simulink model "shipmodel5446"  (Simulink 8.3)
settings: Solver=ode3  StartTime=0.0  StopTime=600  FixedStep=0.3  RelTol=1e-3
libraries: simulink x1
settings Model: Creator=Administrator  LastModifiedBy=hasee
settings OptimizationCC: ExpressionDepthLimit=2147483647
settings DebuggingCC: FcnCallInpInsideContextMsg=UseLocalSettings

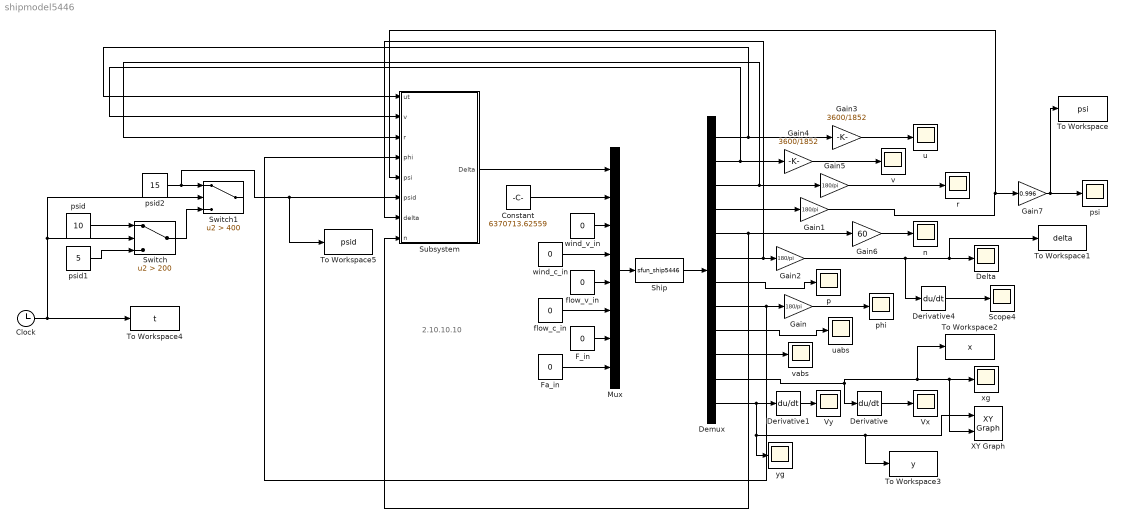
== system shipmodel5446 ==
  note: 2.10.10.10
  Clock : Clock
  Constant : Constant  Value=6370713.62559
  Delta : Scope
      settings: TickLabels=on  TimeRange=600  YMin=-2.5  YMax=25  SaveName=ScopeData5
  Demux : Demux  Outputs=12
  Derivative : Derivative
  Derivative1 : Derivative
  Derivative4 : Derivative
  F_in : Constant  Value=0
  Fa_in : Constant  Value=0
  Gain{,1..2,5} (4 alike) : Gain  Gain=180/pi
  Gain3 : Gain  Gain=3600/1852
  Gain4 : Gain  Gain=3600/1852
  Gain6 : Gain  Gain=60
  Gain7 : Gain  Gain=0.996
  Mux : Mux  Inputs=8
  Scope4 : Scope
      settings: YMin=-3  YMax=3  SaveName=ScopeData18
  Ship : S-Function  FunctionName=sfun_ship5446  EnableBusSupport=off
  Subsystem : Subsystem
  Switch : Switch  Criteria=u2 > Threshold  Threshold=200
  Switch1 : Switch  Criteria=u2 > Threshold  Threshold=400
  To Workspace : ToWorkspace  VariableName=psi  SampleTime=-1
  To Workspace1 : ToWorkspace  VariableName=delta  SampleTime=-1
  To Workspace2 : ToWorkspace  VariableName=x  SampleTime=-1
  To Workspace3 : ToWorkspace  VariableName=y  SampleTime=-1
  To Workspace4 : ToWorkspace  VariableName=t  SampleTime=-1
  To Workspace5 : ToWorkspace  VariableName=psid  SampleTime=-1
  Vx : Scope
      settings: TickLabels=on  SaveName=ScopeData8
  Vy : Scope
      settings: TickLabels=on  SaveName=ScopeData9
  XY Graph : simulink/Sinks/XY Graph  xmin=-2000  xmax=2000  ymin=-200  ymax=4500  st=-1
  flow_c_in : Constant  Value=0
  flow_v_in : Constant  Value=0
  n : Scope
      settings: TickLabels=on  YMin=99.475  YMax=99.8  SaveName=ScopeData4
  p : Scope
      settings: TickLabels=on  SaveName=ScopeData10
  phi : Scope
      settings: YMin=-0.175  YMax=0.125  SaveName=ScopeData11
  psi : Scope
      settings: TickLabels=on  TimeRange=600  YMin=0  YMax=16  SaveName=ScopeData3
  psid : Constant  Value=10
  psid1 : Constant  Value=5
  psid2 : Constant  Value=15
  r : Scope
      settings: TickLabels=on  SaveName=ScopeData2
  u : Scope
      settings: TickLabels=on  YMin=27.45  YMax=28.35
  uabs : Scope
      settings: TickLabels=on  YMin=10.75  YMax=15  SaveName=ScopeData6
  v : Scope
      settings: TickLabels=on  YMin=-0.0975  YMax=-0.055
  vabs : Scope
      settings: TickLabels=on  YMin=-1.75  YMax=0  SaveName=ScopeData7
  wind_c_in : Constant  Value=0
  wind_v_in : Constant  Value=0
  xg : Scope
      settings: TickLabels=on  YMin=250  YMax=475  SaveName=ScopeData12
  yg : Scope
      settings: TickLabels=on  YMin=250  YMax=475  SaveName=ScopeData13
  wires:
  Ship/1 -> Demux/1
  Demux/1 -> Subsystem/1(ut), Gain3/1
  Demux/2 -> Subsystem/2(v), Gain4/1
  Demux/5 -> Subsystem/8(n), Gain6/1
  Demux/6 -> Subsystem/7(delta), Gain2/1
  Demux/7 -> p/1
  Demux/8 -> Subsystem/4(phi), Gain/1
  Gain1/1 -> Subsystem/5(psi), Gain7/1
  Gain/1 -> phi/1
  Gain2/1 -> Derivative4/1, Delta/1, To Workspace1/1
  Gain3/1 -> u/1
  Gain4/1 -> v/1
  Gain5/1 -> r/1
  Gain6/1 -> n/1
  Demux/9 -> uabs/1
  Demux/10 -> vabs/1
  Demux/12 -> Derivative1/1, yg/1, XY Graph/1, To Workspace3/1
  Demux/11 -> Derivative/1, xg/1, XY Graph/2, To Workspace2/1
  Derivative/1 -> Vx/1
  Derivative1/1 -> Vy/1
  wind_v_in/1 -> Mux/3
  wind_c_in/1 -> Mux/4
  flow_v_in/1 -> Mux/5
  F_in/1 -> Mux/7
  Fa_in/1 -> Mux/8
  flow_c_in/1 -> Mux/6
  Mux/1 -> Ship/1
  Constant/1 -> Mux/2
  Derivative4/1 -> Scope4/1
  Demux/4 -> Gain1/1
  Demux/3 -> Subsystem/3(r), Gain5/1
  Subsystem/1(Delta) -> Mux/1
  Clock/1 -> Switch1/2, Switch/2, To Workspace4/1
  psid/1 -> Switch/1
  psid1/1 -> Switch/3
  Switch/1 -> Switch1/3
  psid2/1 -> To Workspace5/1, Subsystem/6(psid), Switch1/1
  Gain7/1 -> psi/1, To Workspace/1

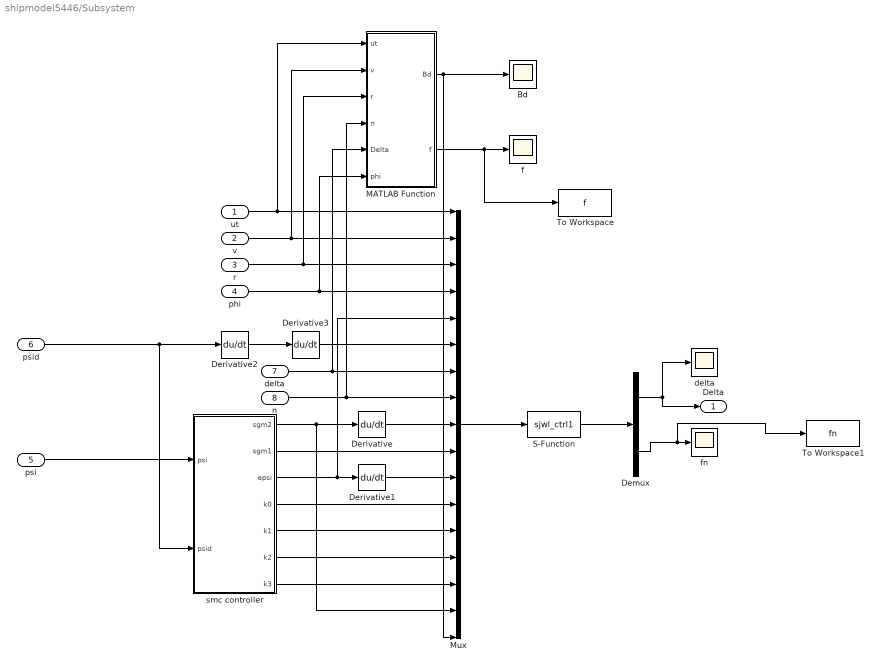
== system shipmodel5446/Subsystem ==
  ut : Inport
  v : Inport  Port=2
  r : Inport  Port=3
  phi : Inport  Port=4
  psi : Inport  Port=5
  psid : Inport  Port=6
  delta : Inport  Port=7
  n : Inport  Port=8
  Bd : Scope
      settings: TickLabels=on  TimeRange=1500  YMin=0.0045  YMax=0.0125  SaveName=ScopeData16
  Demux : Demux  Outputs=2
  Derivative{,1..3} (4 alike) : Derivative
  MATLAB Function : MATLAB Function  TreatAsAtomicUnit=on
  Mux : Mux  Inputs=17
  S-Function : S-Function  FunctionName=sjwl_ctrl1  EnableBusSupport=off
  To Workspace : ToWorkspace  VariableName=f  SampleTime=-1
  To Workspace1 : ToWorkspace  VariableName=fn  SampleTime=-1
  "delta  " : Scope
      settings: TickLabels=on  TimeRange=1500  YMin=-0.25  YMax=-0.235  SaveName=ScopeData14
  f : Scope
      settings: TickLabels=on  TimeRange=600  YMin=-0.0009  YMax=0.0001  SaveName=ScopeData17
  fn : Scope
      settings: TickLabels=on  TimeRange=600  YMin=6.64e-06  YMax=6.83e-06  SaveName=ScopeData15
  smc controller : Subsystem
  Delta : Outport
  wires:
  psi/1 -> smc controller/1(psi)
  psid/1 -> smc controller/2(psid), Derivative2/1
  ut/1 -> MATLAB Function/1(ut), Mux/1
  v/1 -> MATLAB Function/2(v), Mux/2
  r/1 -> MATLAB Function/3(r), Mux/3
  phi/1 -> MATLAB Function/6(phi), Mux/4
  delta/1 -> MATLAB Function/5(Delta), Mux/7
  Mux/1 -> S-Function/1
  S-Function/1 -> Demux/1
  Demux/1 -> Delta/1, "delta  "/1
  Demux/2 -> To Workspace1/1, fn/1
  smc controller/1(sgm2) -> Mux/16, Derivative/1
  smc controller/7(k3) -> Mux/15
  smc controller/6(k2) -> Mux/14
  smc controller/5(k1) -> Mux/13
  smc controller/4(k0) -> Mux/12
  Derivative/1 -> Mux/9
  Derivative1/1 -> Mux/11
  smc controller/3(epsi) -> Derivative1/1, Mux/5
  smc controller/2(sgm1) -> Mux/10
  n/1 -> MATLAB Function/4(n), Mux/8
  Derivative2/1 -> Derivative3/1
  Derivative3/1 -> Mux/6
  MATLAB Function/1(Bd) -> Mux/17, Bd/1
  MATLAB Function/2(f) -> To Workspace/1, f/1

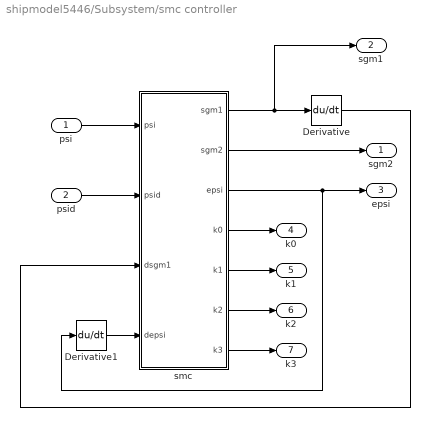
== system shipmodel5446/Subsystem/smc controller ==
  psi : Inport
  psid : Inport  Port=2
  Derivative : Derivative
  Derivative1 : Derivative
  "smc " : MATLAB Function  TreatAsAtomicUnit=on
  sgm2 : Outport
  sgm1 : Outport  Port=2
  epsi : Outport  Port=3
  k0 : Outport  Port=4
  k1 : Outport  Port=5
  k2 : Outport  Port=6
  k3 : Outport  Port=7
  wires:
  "smc "/1(sgm1) -> sgm1/1, Derivative/1
  Derivative/1 -> "smc "/3(dsgm1)
  psi/1 -> "smc "/1(psi)
  psid/1 -> "smc "/2(psid)
  "smc "/2(sgm2) -> sgm2/1
  "smc "/3(epsi) -> Derivative1/1, epsi/1
  Derivative1/1 -> "smc "/4(depsi)
  "smc "/4(k0) -> k0/1
  "smc "/5(k1) -> k1/1
  "smc "/6(k2) -> k2/1
  "smc "/7(k3) -> k3/1

== matlab function Subsystem/smc controller/smc  ==
  data: psi input double; psid input double; dsgm1 input double; sgm1 output double; sgm2 output double; epsi output double; depsi input double; k0 output double; k1 output double; k2 output double; k3 output double
function [sgm1,sgm2,epsi,k0,k1,k2,k3]= fcn(psi,psid,dsgm1,depsi)
%#codegen

% k0=0.04;k1=5;k2=0.03;k3=8;
% k0=0.1;k1=0.3;k2=0.1;k3=0.1;
%  k0=0.01;k1=8;k2=0.1;k3=10;
k0=0.04;k1=5;k2=0.1;k3=9;


epsi=psid-psi;

% k1=0.2;k3=1;m=3;
sgm1=k1*tanh(k0*epsi)+depsi;
sgm2=k3*tanh(k2*sgm1)+dsgm1;

% sgm1=k1*(epsi^(2*m-1))+depsi;
% sgm2=k3*(sgm1^(2*m-1))+dsgm1;

== matlab function Subsystem/MATLAB Function ==
  data: ut input double; v input double; r input double; n input double; Delta input double; phi input double; Bd output double; f output double
%%%%%%%%%%%%%%%%%%%%%%%%%%%%%%%%%%%%%%%%%%%%%%%%%%%%%%%%%%%%%
%%源自: 沈智鹏 著《船舶运动自适应滑模控制》 2019年科学出版社
%%下载地址www.shenbert.cn/book/shipmotionASMC.html
%%%%%%%%%%%%%%%%%%%%%%%%%%%%%%%%%%%%%%%%%%%%%%%%%%%%%%%%%%%%%%
function [Bd,f] = fcn(ut,v,r,n,Delta,phi)
V=sqrt(ut*ut+v*v);%u=x(1) v=x(2)
        da=10.5;%9.34+0.25;%尾吃水13.8;%12.5;%
	  df=7.5;%4.97+0.25;%首吃水14.3;%13.8;%
	  Dh=9.0;%舵高s   ;%11.411.4;;%+7.00+0.25
      pa=1.205;%%%**空气密度
      Lpp=267.0;%船长
	  B=39.8;%船宽
	  Db=6.466;%舵宽
      P=9.657;%da螺距
      luow=1026;%小luow是密度 水密度
      Dp=9.2;%螺旋桨直径
      Ds=23.6;%型深
      d=(da+df)/2;%吃水
      m=(165.89*d*d + 4383.9*d)*1000;%排水量
      Cb=m/(Lpp*B*d*1.025*1000);
      AR=(d-7.41)/(12.5-7.41)*(81.44-43.14)+43.14;%舵叶面积 
	  d_B=d/B;L_B=Lpp/B;
	  mx=m/100*(0.398+11.97*Cb*(1+3.73*d_B)-2.89*Cb*L_B*(1+1.13*d_B)+0.175*Cb*L_B*L_B*(1+0.541*d_B)-1.107*L_B*d_B); 
	  my=m*(0.882-0.54*Cb*(1-1.6*d_B)-0.156*L_B*(1-0.673*Cb)+0.826*d_B*L_B*(1-0.678*d_B)-0.638*Cb*d_B*L_B*(1-0.669*d_B)); 
      wp0=0.5*Cb-0.05;   
      fa=6.13*Dh/Db/(2.25+Dh/Db);
      gma=-22.2*(Cb*B/Lpp)*(Cb*B/Lpp)+0.02*(Cb*B/Lpp)+0.68; 
      gmaR=1.1633-1.98828*Cb+1.3902*Cb*Cb;
      tR=0.7382-0.0539*Cb+0.1755*Cb*Cb; 
      ifaH=0.6784-1.3374*Cb+1.8891*Cb*Cb;
	  xH=-(0.4+0.1*Cb)*Lpp;
      xR=-0.5*Lpp;
      xb=1.87;
	  Jzz=1/100.0*(33-76.85*Cb*(1-0.784*Cb)+3.43*L_B*(1-0.63*Cb))*Lpp*Lpp;
      Izz=(1.0+(Cb^4.5))*m*(Lpp*Lpp+power(B,2.4))/24.0;
      lmd=2.0*d/Lpp; 
      CbBL=Cb*B/Lpp;
      CbdB=(1-Cb)*d_B;
      tao=(da-df)/d;
      lg_mass=1/2.0*luow*Lpp*Lpp*d;
      Yv=-(pi/2.0*lmd+1.4*CbBL)*(1+(25.0*CbBL-2.25)*tao);
      Yr=((m+mx)/lg_mass-1.5*CbBL)*(1+(571*CbdB*CbdB-81*d*(1-Cb)/B+2.1)*tao);
      Yvrr=(-5.95*CbdB)*(1+(40*CbdB-2)*tao);
      Yvvr=(1.5*Cb*d_B-0.65)*(1+(110*CbdB-9.7)*tao);
      Nv=-lmd*(1.0-tao);
      Nr=-(0.54*lmd-lmd*lmd)*(1+(34*CbBL-3.4)*tao);
      Nvv=0.5*luow*Lpp*Lpp*d*(0.96*CbdB-0.066)*(1+(58*CbdB-5)*tao);
      Nrr=0.5*luow*Lpp*Lpp*Lpp*Lpp*d*(0.5*CbBL-0.09)*(1-(30*CbBL-2.6)*tao);
      Nvrr=(0.5*CbBL-0.05)*(1+(48*(CbBL^2)-16*CbBL+1.3)*100*tao);
      Nvvr=(-57.5*(CbBL^2)+18.4*CbBL-1.6)*(1+(3*CbBL-1)*tao);
      Nv1=0.5*luow*Lpp*Lpp*d*V*Nv;
      Nr1=0.5*luow*Lpp*Lpp*Lpp*d*V*Nr;
      Nvrr1=0.5*luow*Lpp*Lpp*Lpp*Lpp*d/V*Nvrr;
      Nvvr1=0.5*luow*Lpp*Lpp*Lpp*d/V*Nvvr;
    Yv1=0.5*luow*Lpp*d*V*Yv;	  
    Yr1=0.5*luow*Lpp*Lpp*d*V*Yr;   
    Yvrr1=0.5*luow*Lpp*Lpp*Lpp*d/V*Yvrr;
    Yvvr1=0.5*luow*Lpp*Lpp*d/V*Yvvr;
    Yvv=0.5*luow*Lpp*d*((-2.5*(1-Cb)*B/(d-0.5))*(1-(35.7*CbBL-2.5)*tao));
    Yrr=0.5*luow*Lpp*Lpp*Lpp*d*((0.343*Cb*d_B-0.07)*(1+(45*CbBL-8.1)*tao));
    Nphi=1/2.0*luow*Lpp*d*V*V*(-0.008);
    Nvphi=1/2.0*luow*Lpp*d*V*(1.72*Nv);
    Nrphi=1/2.0*luow*Lpp*d*V*V*(-2.6*Nr);
    
    m33=Izz+Jzz;


     beta=atan2((-v),(ut));%u=x(1) v=x(2)
	 betap=beta+0.5*r*Lpp/V;%r=x(3) 
     betaR=beta+r*Lpp/V;
     wp=wp0*exp(-4.0*betap*betap);
    up=(1.0-wp)*ut;%u=x(1)
    s=1.0-up/n/P;% n=x(5)
    eta=Dp/Dh;

    k=0.6;
    Gs=eta*k*(2.0-(2.0-k)*s)*s/(1.0-s)/(1.0-s); 
    s0=1-(1-wp0)*ut/n/P;% n=x(5)u=x(1)
    delt0=-s0/57.3;
    
    if(Delta<0)  
        K=1.065;
    else
        K=0.935;
    end
   
    uR=up*(1+K*Gs)^0.5; 
    vRp=uR*delt0;
    vR=vRp-gmaR*(v-Lpp*r);%r=x(3)v=x(2)
    UR2=uR*uR+vR*vR;
    J=ut*(1-wp)/n/Dp;%u=x(1)  n=x(5)
    if(J<=0.3)
        L_ifaH=ifaH*J/0.3;% p137, 3-5-119   
    else
        L_ifaH=ifaH;
    end

Bd=(-1.0/2.0)*(xR+L_ifaH*xH)*luow*AR*fa*UR2*cos(Delta)/(m33);
xC=xb;
YH=Yv1*v+Yr1*r+Yvv*abs(v)*v+Yrr*abs(r)*r+Yvvr1*v*v*r+Yvrr1*v*r*r;
L_NH0=Nv1*v+Nr1*r+Nvv*abs(v)*v+Nrr*abs(r)*r+Nvvr1*v*v*r+Nvrr1*v*r*r;
L_NH1=Nphi*phi+Nvphi*v*abs(phi)+Nrphi*r*abs(phi);
NH=L_NH0+L_NH1;
f=(NH-YH*xC)/(m33);
